simulink model "WEEK1_QN3"  (R2020b)
settings: Solver=VariableStepAuto  StartTime=0.0  StopTime=1.0  MaxStep=0.001  RelTol=1e-3
settings Model: Creator=dell  LastModifiedBy=dell

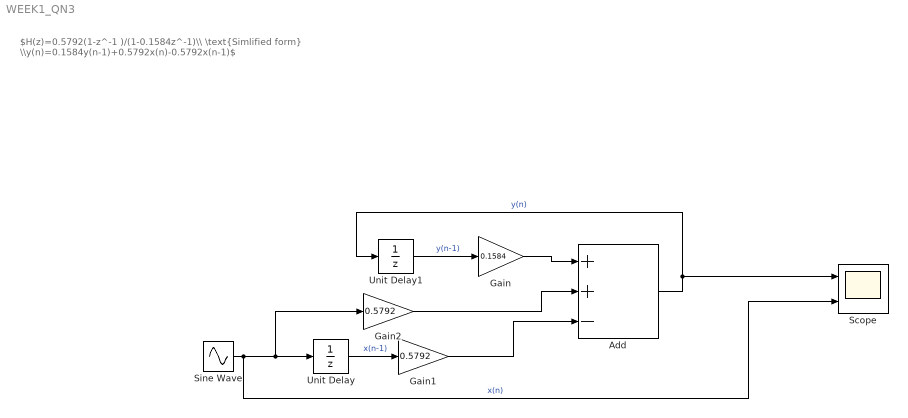
== system WEEK1_QN3 ==
  note: $H(z)=0.5792(1-z^-1 )/(1-0.1584z^-1)\\ \text{Simlified form} \\y(n)=0.1584y(n-1)+0.5792x(n)-0.5792x(n-1)$
  Add : Sum  Inputs=++-
  Gain : Gain  Gain=0.1584
  Gain1 : Gain  Gain=0.5792
  Gain2 : Gain  Gain=0.5792
  Scope : Scope  NumInputPorts=2
  Sine Wave : Sin  Frequency=400  SampleTime=0
  Unit Delay : UnitDelay  SampleTime=-1  HasFrameUpgradeWarning=on
  Unit Delay1 : UnitDelay  SampleTime=-1  HasFrameUpgradeWarning=on
  wires:
  Add/1 -> Scope/1, Unit Delay1/1  "y(n)"
  Unit Delay1/1 -> Gain/1  "y(n-1)"
  Gain/1 -> Add/1
  Sine Wave/1 -> Scope/2, Gain2/1, Unit Delay/1  "x(n)"
  Unit Delay/1 -> Gain1/1  "x(n-1)"
  Gain1/1 -> Add/3
  Gain2/1 -> Add/2
